simulink model "funciones_de_transferencia_con_ceros"  (Simulink 7.7)
settings: Solver=ode3  StartTime=0.0  StopTime=20.0  FixedStep=0.01  MaxStep=0.01  MinStep=0.01  RelTol=0.001  AbsTol=0.001
settings Model: Creator=juen  LastModifiedBy=juen
settings SolverCC: InitialStep=0.01
settings DataIOCC: LimitDataPoints=off  SaveFormat=StructureWithTime

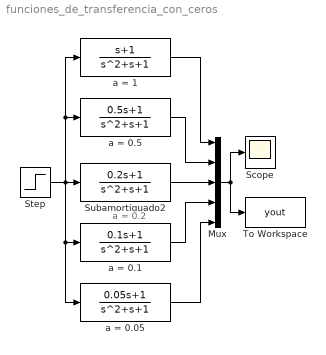
== system funciones_de_transferencia_con_ceros ==
  note: a = 0.2
  Mux : Mux  Inputs=5
  Scope : Scope
  Step : Step  SampleTime=0
  Subamortiguado2 : TransferFcn  Numerator=[0.2 1]  Denominator=[1 1 1]
  To Workspace : ToWorkspace  VariableName=yout  SampleTime=-1  SaveFormat=Structure With Time
  a = 0.05 : TransferFcn  Numerator=[0.05 1]  Denominator=[1 1 1]
  a = 0.1 : TransferFcn  Numerator=[0.1 1]  Denominator=[1 1 1]
  a = 0.5 : TransferFcn  Numerator=[0.5 1]  Denominator=[1 1 1]
  a = 1 : TransferFcn  Numerator=[1 1]  Denominator=[1 1 1]
  wires:
  Subamortiguado2/1 -> Mux/3
  a = 0.1/1 -> Mux/4
  a = 0.05/1 -> Mux/5
  Mux/1 -> To Workspace/1, Scope/1
  a = 0.5/1 -> Mux/2
  a = 1/1 -> Mux/1
  Step/1 -> a = 0.1/1, a = 0.05/1, Subamortiguado2/1, a = 0.5/1, a = 1/1
